simulink model "erziyoudu2017"  (R2017b)
settings: Solver=VariableStepAuto  StartTime=0.0  StopTime=10.0  RelTol=1e-3
undefined symbols (not defined in the file or in its folder): alpha, DIST_FR_AXLE_TO_CG_NVV, DIST_RE_AXLE_TO_CG_NVV, Fy, Fz, VEHICLE_MASS_NVV, VEHICLE_YAW_INERTIA_NVV
libraries: simulink x3, simulink_extras x2
settings Model: Creator=Ecoking  LastModifiedBy=Ecoking
settings DataIOCC: ReturnWorkspaceOutputs=on
settings DebuggingCC: UnconnectedInputMsg=none  UnconnectedOutputMsg=none  UnconnectedLineMsg=none
settings ModelReferenceCC: EnableRefExpFcnMdlSchedulingChecks=off
settings SFSimCC: SimUseLocalCustomCode=on
settings RTWCC: Description=Generic Real-Time Target  RTWUseLocalCustomCode=on

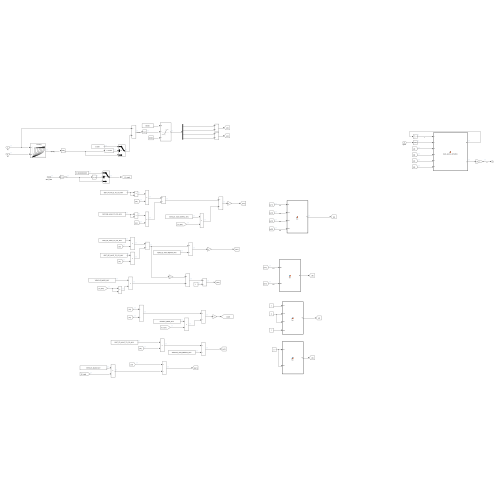
[thumbnail: Simulink's stored preview of the top-level diagram]
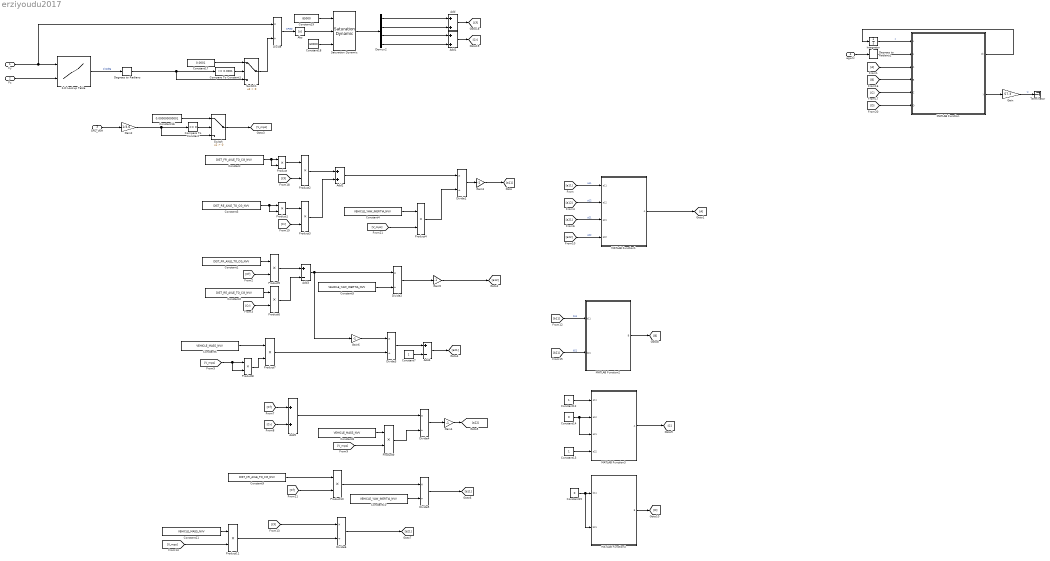
== system erziyoudu2017 ==
  Fy : Inport
  Fz : Inport  Port=2
  SPD_VEH : Inport  Port=3
  agwhl : Inport  Port=4
  2-D Lookup Table : Lookup_n-D  BreakpointsForDimension1=Fy  BreakpointsForDimension2=Fz  Table=alpha  InternalRulePriority=Speed  RndMeth=Simplest  InputSameDT=on
  Abs : Abs
  Add{,1..2,5} (4 alike) : Sum
  Add3 : Sum  Inputs=+-
  Add4 : Sum  Inputs=+-
  Compare To Constant : simulink/Logic and Bit Operations/Compare To Constant  relop===  const=0  OutDataTypeStr=boolean
  Compare To Constant1 : simulink/Logic and Bit Operations/Compare To Constant  relop=<=  const=0.0001  OutDataTypeStr=boolean
  Constant : Constant  Value=DIST_FR_AXLE_TO_CG_NVV
  Constant1 : Constant  Value=DIST_FR_AXLE_TO_CG_NVV
  Constant10 : Constant  Value=VEHICLE_YAW_INERTIA_NVV
  Constant11 : Constant  Value=VEHICLE_MASS_NVV
  Constant12 : Constant
  Constant13 : Constant
  Constant14 : Constant  Value=0
  Constant15 : Constant  Value=0
  Constant16 : Constant  Value=0.000000000001
  Constant17 : Constant  Value=0.0001
  Constant18 : Constant  Value=60000
  Constant19 : Constant  Value=85000
  Constant2 : Constant  Value=DIST_RE_AXLE_TO_CG_NVV
  Constant3 : Constant  Value=DIST_RE_AXLE_TO_CG_NVV
  Constant4 : Constant  Value=VEHICLE_YAW_INERTIA_NVV
  Constant5 : Constant  Value=VEHICLE_YAW_INERTIA_NVV
  Constant6 : Constant  Value=VEHICLE_MASS_NVV
  Constant7 : Constant
  Constant8 : Constant  Value=VEHICLE_MASS_NVV
  Constant9 : Constant  Value=DIST_FR_AXLE_TO_CG_NVV
  Degrees to Radians : simulink_extras/Transformations/Degrees to Radians
  Degrees to Radians1 : simulink_extras/Transformations/Degrees to Radians
  Demux2 : Demux
  Divide{,1..6} (7 alike) : Product  Inputs=*/
  Gain : Gain  Gain=57.3
  Gain2 : Gain  Gain=1/3.6
  Gain{3..6} (4 alike) : Gain  Gain=-1
  Integrator : Integrator  InitialCondition=[0;0]
  MATLAB Function : MATLAB Function  TreatAsAtomicUnit=on
  MATLAB Function1 : MATLAB Function  TreatAsAtomicUnit=on
  MATLAB Function2 : MATLAB Function  TreatAsAtomicUnit=on
  MATLAB Function3 : MATLAB Function  TreatAsAtomicUnit=on
  MATLAB Function4 : MATLAB Function  TreatAsAtomicUnit=on
  Product{,1..11} (12 alike) : Product
  Saturation Dynamic : simulink/Discontinuities/Saturation Dynamic  OutMin=[]  OutMax=[]  OutDataTypeStr=Inherit: Same as second input  OutDataType=fixdt(1, 16)  OutScaling=2^-10  DoSatur=off
  Switch : Switch  Criteria=u2 > Threshold
  Switch1 : Switch  Criteria=u2 > Threshold
  Terminator : Terminator
  wires:
  Constant19/1 -> Saturation Dynamic/1
  Constant18/1 -> Saturation Dynamic/3
  Gain5/1 -> [a12]
  Constant9/1 -> Product10/1
  Gain4/1 -> [a22]
  agwhl/1 -> Degrees to Radians1/1
  Abs/1 -> Saturation Dynamic/2
  Gain6/1 -> Divide3/1
  Gain/1 -> Terminator/1  "w"
  Gain3/1 -> [a11]
  Add/1 -> [Cf]
  Add1/1 -> [Cr]
  Degrees to Radians/1 -> Compare To Constant1/1, Switch1/3
  Switch1/1 -> Divide/2
  Constant17/1 -> Switch1/1
  Saturation Dynamic/1 -> Demux2/1
  Product4/1 -> Divide1/2
  Gain2/1 -> Switch/3, Compare To Constant/1
  Divide6/1 -> [b21]
  Divide/1 -> Abs/1  "CPGD"
  [V_mps] -> Product4/2
  Constant16/1 -> Switch/1
  Compare To Constant/1 -> Switch/2
  Add3/1 -> Gain6/1, Divide2/1
  [D] -> MATLAB Function/6(D)
  Product7/1 -> Divide3/2
  [C] -> MATLAB Function/5(C)
  [b11] -> MATLAB Function2/1(b11)  "b11"
  [Cf] -> Product10/2
  [Cr] -> Add5/2
  [V_mps] -> Product11/2
  Constant11/1 -> Product11/1
  Constant12/1 -> MATLAB Function3/1(a11)
  [a21] -> MATLAB Function1/3(a21)  "a21"
  Divide3/1 -> Add4/1
  [Cf] -> Divide6/1
  Product11/1 -> Divide6/2
  [B] -> MATLAB Function/4(B)
  Divide4/1 -> Gain4/1
  Switch/1 -> [V_mps]
  Product10/1 -> Divide5/1
  [V_mps] -> Product9/2
  Divide5/1 -> [b11]
  Constant14/1 -> MATLAB Function3/3(a21), MATLAB Function3/2(a12)
  Add5/1 -> Divide4/1
  Constant8/1 -> Product9/1
  [Cf] -> Add5/1
  Constant13/1 -> MATLAB Function3/4(a22)
  Divide2/1 -> Gain5/1
  [a22] -> MATLAB Function1/4(a22)  "a22"
  MATLAB Function2/1(B) -> [B]
  Constant7/1 -> Add4/2
  [a12] -> MATLAB Function1/2(a12)  "a12"
  Constant2/1 -> Product6/1
  Add4/1 -> [a21]
  [Cr] -> Product6/2
  Product9/1 -> Divide4/2
  MATLAB Function/1(dx) -> Integrator/1
  SPD_VEH/1 -> Gain2/1
  Constant1/1 -> Product5/1
  Constant3/1 -> Product1/2, Product1/1
  Product3/1 -> Add2/2
  Fy/1 -> Divide/1, 2-D Lookup Table/1
  Constant10/1 -> Divide5/2
  Constant15/1 -> MATLAB Function4/2(b21), MATLAB Function4/1(b11)
  Product2/1 -> Add2/1
  Constant/1 -> Product/2, Product/1
  [Cf] -> Product5/2
  Integrator/1 -> MATLAB Function/1(x)  "x"
  Product/1 -> Product2/1
  [Cr] -> Product3/2
  Constant6/1 -> Product7/1
  [A] -> MATLAB Function/3(A)
  Compare To Constant1/1 -> Switch1/2
  Product1/1 -> Product3/1
  Demux2/3 -> Add1/1
  Add2/1 -> Divide1/1
  Constant4/1 -> Product4/1
  [b21] -> MATLAB Function2/2(b21)  "b21"
  MATLAB Function1/1(A) -> [A]
  Divide1/1 -> Gain3/1
  [Cf] -> Product2/2
  MATLAB Function4/1(B) -> [D]
  Demux2/4 -> Add1/2
  Demux2/1 -> Add/1
  2-D Lookup Table/1 -> Degrees to Radians/1  "slipdeg"
  Degrees to Radians1/1 -> MATLAB Function/2(u)
  Product6/1 -> Add3/2
  Fz/1 -> 2-D Lookup Table/2
  Demux2/2 -> Add/2
  Constant5/1 -> Divide2/2
  [a11] -> MATLAB Function1/1(a11)  "a11"
  [V_mps] -> Product8/2, Product8/1
  MATLAB Function3/1(A) -> [C]
  MATLAB Function/2(y) -> Gain/1
  Product5/1 -> Add3/1
  Product8/1 -> Product7/2

== matlab function erziyoudu2017/MATLAB Function1 ==
  data: a11 input; A output; a12 input; a21 input; a22 input
function A = fcn(a11, a12, a21, a22)
%#codegen
A = [a11, a12; a21, a22];
end

== matlab function erziyoudu2017/MATLAB Function ==
  data: x input; dx output; u input; y output; A input; B input; C input; D input
function [dx, y] = state_space_derivative(x, u, A, B, C, D)
    % 计算连续时间状态导数
    dx = A * x + B * u;
    y  = C * x + D * u;
end

== matlab function erziyoudu2017/MATLAB Function2 ==
  data: b11 input; B output; b21 input
function B = fcn(b11, b21)
%#codegen
B = [b11;b21];
end

== matlab function erziyoudu2017/MATLAB Function3 ==
  data: a11 input; A output; a12 input; a21 input; a22 input
function A = fcn(a11, a12, a21, a22)
%#codegen
A = [a11, a12; a21, a22];
end

== matlab function erziyoudu2017/MATLAB Function4 ==
  data: b11 input; B output; b21 input
function B = fcn(b11, b21)
%#codegen
B = [b11;b21];
end
